simulink library "SafetyCheckerSOMANET"  (R2016b)
settings: Solver=VariableStepAuto  StartTime=0.0  StopTime=10.0  RelTol=1e-3
undefined symbols (not defined in the file or in its folder): SomanetError
libraries: simulink x1, I2tChecker x1, EndStopChecker x1, PhaseCurrentsChecker x1, TemperatureChecker x1, TimestampChecker x1, TorqueChecker x1
settings Model: Creator=Nathan  LastModifiedBy=RKFE

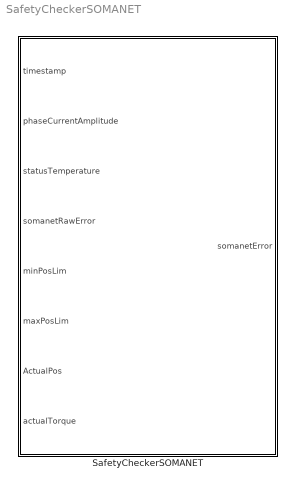
== system SafetyCheckerSOMANET ==
  SafetyCheckerSOMANET : Subsystem

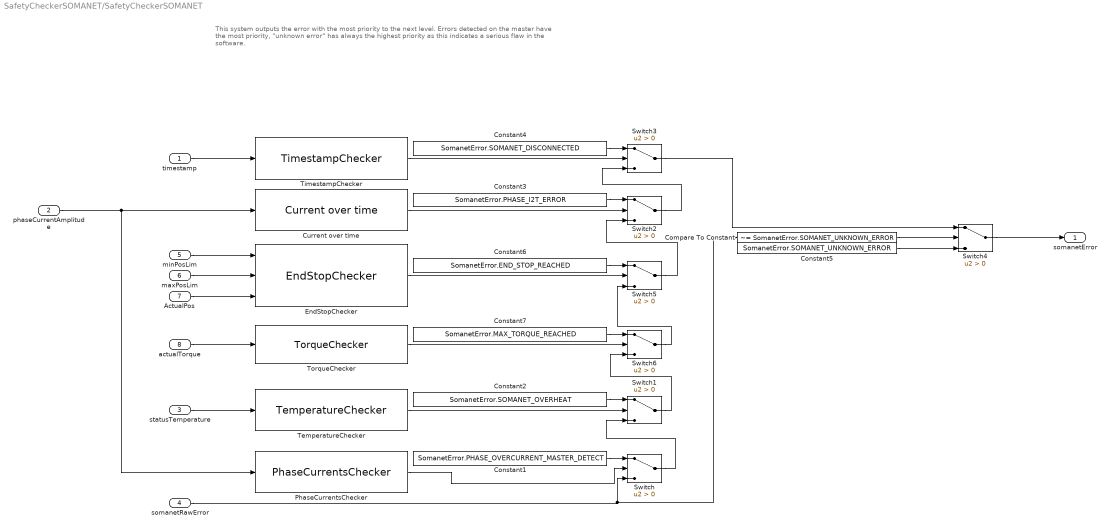
== system SafetyCheckerSOMANET/SafetyCheckerSOMANET ==
  note: This system outputs the error with the most priority to the next level.
      | Errors detected on the master have the most priority, "unknown error" has always the highest priority as this indicates a serious flaw in the software.
  timestamp : Inport  BusOutputAsStruct=on
  phaseCurrentAmplitude : Inport  Port=2
  statusTemperature : Inport  Port=3  BusOutputAsStruct=on
  somanetRawError : Inport  Port=4
  minPosLim : Inport  Port=5
  maxPosLim : Inport  Port=6
  ActualPos : Inport  Port=7
  actualTorque : Inport  Port=8
  Compare To Constant : simulink/Logic and Bit Operations/Compare To Constant  relop=~=  const=SomanetError.SOMANET_UNKNOWN_ERROR  OutDataTypeStr=boolean
  Constant1 : Constant  Value=SomanetError.PHASE_OVERCURRENT_MASTER_DETECT
  Constant2 : Constant  Value=SomanetError.SOMANET_OVERHEAT
  Constant3 : Constant  Value=SomanetError.PHASE_I2T_ERROR
  Constant4 : Constant  Value=SomanetError.SOMANET_DISCONNECTED
  Constant5 : Constant  Value=SomanetError.SOMANET_UNKNOWN_ERROR
  Constant6 : Constant  Value=SomanetError.END_STOP_REACHED
  Constant7 : Constant  Value=SomanetError.MAX_TORQUE_REACHED
  Current over time : I2tChecker/Current over time
  EndStopChecker : EndStopChecker/EndStopChecker
  PhaseCurrentsChecker : PhaseCurrentsChecker/PhaseCurrentsChecker
  Switch{,1..6} (7 alike) : Switch  Criteria=u2 > Threshold
  TemperatureChecker : TemperatureChecker/TemperatureChecker
  TimestampChecker : TimestampChecker/TimestampChecker
  TorqueChecker : TorqueChecker/TorqueChecker
  somanetError : Outport
  wires:
  Switch4/1 -> somanetError/1
  PhaseCurrentsChecker/1 -> Switch/2
  Constant1/1 -> Switch/1
  Switch/1 -> Switch1/3
  TemperatureChecker/1 -> Switch1/2
  Current over time/1 -> Switch2/2
  TimestampChecker/1 -> Switch3/2
  Constant2/1 -> Switch1/1
  Constant3/1 -> Switch2/1
  Constant4/1 -> Switch3/1
  Switch2/1 -> Switch3/3
  somanetRawError/1 -> Switch/3, Compare To Constant/1
  Switch3/1 -> Switch4/1
  Compare To Constant/1 -> Switch4/2
  Constant5/1 -> Switch4/3
  timestamp/1 -> TimestampChecker/1
  phaseCurrentAmplitude/1 -> PhaseCurrentsChecker/1, Current over time/1
  statusTemperature/1 -> TemperatureChecker/1
  ActualPos/1 -> EndStopChecker/3
  maxPosLim/1 -> EndStopChecker/2
  minPosLim/1 -> EndStopChecker/1
  Constant6/1 -> Switch5/1
  Switch5/1 -> Switch2/3
  actualTorque/1 -> TorqueChecker/1
  TorqueChecker/1 -> Switch6/2
  Constant7/1 -> Switch6/1
  Switch1/1 -> Switch6/3
  EndStopChecker/1 -> Switch5/2
  Switch6/1 -> Switch5/3
